simulink library "rtlsdr_book_library"  (R2014b)
settings: Solver=ode45  StartTime=0.0  StopTime=10.0  RelTol=1e-3
values from neighbouring files (symbols this model uses):
  frm = rmfield(frm , 'master_frame')    [image_frame_gen.m]    (also in import_rtlsdr_data.m = cast(frm,obj.data_type))
  src = rmfield(src , 'master_time')    [ASCII_frame_gen.m]
undefined symbols (not defined in the file or in its folder): den, dfilt, fdesignblkfcn, gcbh, iir, num, rtlsdr_frmsize, rtlsdr_fs
undefined symbols (not defined in the file): costas
libraries: dspsigops x6, commsynccomp2 x4, dspsrcs4 x2, dspstat3 x2, dspobslib x2, simulink_extras x2, dspmtrx3 x2, dsparch4 x1, rtlsdr_book_library x1, dspspect3 x1, commrflib2 x1
(part 3 of 5)

== system rtlsdr_book_library/Sync Tools for Analogue Comms/Phase Locked Loop Demodulator/Reduce Output Rate ==
  in : Inport
  Clock : simulink_extras/Flip Flops/Clock  period=1/rate*2
  Delay : Delay  DelayLength=1  InitialCondition=0
  Enabled Subsystem : Subsystem  TreatAsAtomicUnit=on
  XOR : Logic  Operator=XOR  IconShape=distinctive  AllPortsSameDT=off  OutDataTypeStr=boolean
  out : Outport
  wires:
  in/1 -> Enabled Subsystem/1(In1)
  Enabled Subsystem/1(Out1) -> out/1
  XOR/1 -> Enabled Subsystem/Enable
  Clock/1 -> Delay/1, XOR/1
  Delay/1 -> XOR/2

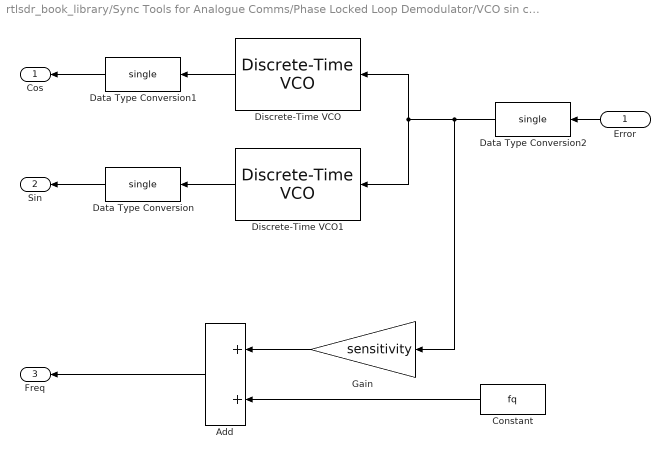
== system rtlsdr_book_library/Sync Tools for Analogue Comms/Phase Locked Loop Demodulator/VCO sin cos ==
  Error : Inport
  Add : Sum
  Constant : Constant  Value=fq  OutDataTypeStr=single  SampleTime=1/fs
  Data Type Conversion : DataTypeConversion  OutDataTypeStr=single
  Data Type Conversion1 : DataTypeConversion  OutDataTypeStr=single
  Data Type Conversion2 : DataTypeConversion  OutDataTypeStr=single
  Discrete-Time VCO : commsynccomp2/Discrete-Time VCO  Ac=1  Fc=fq  Kc=sensitivity  Ph=pi/2  ts=1/fs
  Discrete-Time VCO1 : commsynccomp2/Discrete-Time VCO  Ac=1  Fc=fq  Kc=sensitivity  Ph=0  ts=1/fs
  Gain : Gain  Gain=sensitivity
  Cos : Outport
  Sin : Outport  Port=2
  Freq : Outport  Port=3
  wires:
  Discrete-Time VCO1/1 -> Data Type Conversion/1
  Discrete-Time VCO/1 -> Data Type Conversion1/1
  Error/1 -> Data Type Conversion2/1
  Gain/1 -> Add/1
  Constant/1 -> Add/2
  Add/1 -> Freq/1
  Data Type Conversion/1 -> Sin/1
  Data Type Conversion1/1 -> Cos/1
  Data Type Conversion2/1 -> Gain/1, Discrete-Time VCO1/1, Discrete-Time VCO/1
